simulink model "ten"  (R2020a)
settings: Solver=VariableStepAuto  StartTime=0.0  StopTime=500  RelTol=1e-3
settings Model: Creator=ggski  LastModifiedBy=ggski

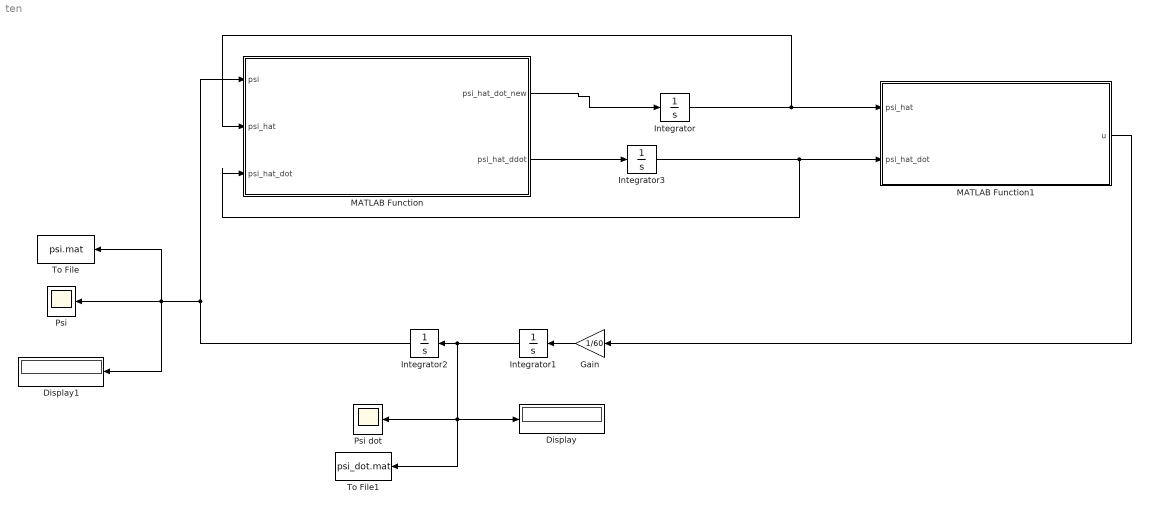
== system ten ==
  Display : Display
  Display1 : Display
  Gain : Gain  Gain=1/60
  Integrator : Integrator
  Integrator1 : Integrator  InitialCondition=0.1
  Integrator2 : Integrator
  Integrator3 : Integrator
  MATLAB Function : MATLAB Function  TreatAsAtomicUnit=on
  MATLAB Function1 : MATLAB Function  TreatAsAtomicUnit=on
  Psi : Scope
  Psi dot : Scope
  To File : ToFile  Filename=psi.mat  MatrixName=psi
  To File1 : ToFile  Filename=psi_dot.mat  MatrixName=psi_dot
  wires:
  MATLAB Function/1(psi_hat_dot_new) -> Integrator/1
  MATLAB Function1/1(u) -> Gain/1
  Gain/1 -> Integrator1/1
  MATLAB Function/2(psi_hat_ddot) -> Integrator3/1
  Integrator/1 -> MATLAB Function/2(psi_hat), MATLAB Function1/1(psi_hat)
  Integrator3/1 -> MATLAB Function/3(psi_hat_dot), MATLAB Function1/2(psi_hat_dot)
  Integrator1/1 -> Integrator2/1, To File1/1, Display/1, Psi dot/1
  Integrator2/1 -> To File/1, Psi/1, Display1/1, MATLAB Function/1(psi)

== matlab function ten/MATLAB Function1 ==
  data: psi_hat input; u output; psi_hat_dot input
function u = the_u(psi_hat, psi_hat_dot)
K_p = 60;
K_d = 60;
u = -K_p*psi_hat - K_d*psi_hat_dot;

end

== matlab function ten/MATLAB Function ==
  data: psi input; psi_hat_dot_new output; psi_hat input; psi_hat_dot input; psi_hat_ddot output
function [psi_hat_dot_new, psi_hat_ddot]= ten(psi, psi_hat, psi_hat_dot)
K_p = 60;
K_d = 60;
L1 = 50;
L2 = 50;
temp = [0, 1; -K_p, -K_d]*[psi_hat; psi_hat_dot]+[L1; L2]*(psi-psi_hat);
psi_hat_dot_new = temp(1);
psi_hat_ddot = temp(2);
end
